simulink model "common_2"  (R2018b)
settings: Solver=ode4  StartTime=0.0  StopTime=tmax  FixedStep=0.005  RelTol=1e-3  EnableMultiTasking=on
values from neighbouring files (symbols this model uses):
  dq_init = [0.01 0.01]    [paraInit.m]
  g = 9.81    [paraInit.m]
  q_init = [0.01 0.01]    [paraInit.m]
undefined symbols (not defined in the file or in its folder): para
settings Model: Creator=Administrator  LastModifiedBy=q5461
settings DataIOCC: LimitDataPoints=on
settings OptimizationCC: LifeSpan=inf
settings DebuggingCC: AllowSymbolicDim=off  SFUnexpectedBacktrackingDiag=warning  SFNoUnconditionalDefaultTransitionDiag=warning  SFExecutionAtInitializationDiag=none
settings ModelReferenceCC: PropagateSignalLabelsOutOfModel=off
settings SFSimCC: SimUseLocalCustomCode=off
settings RTWCC: RTWUseLocalCustomCode=off
settings CodeAppCC: StateflowObjectComments=on
settings GRTTargetCC: TargetLangStandard=C89/C90 (ANSI)
settings ConfigComp: CovMetricSettings=dw  CovHtmlReporting=on  CovSaveCumulativeToWorkspaceVar=on  CovSaveSingleToWorkspaceVar=on  CovExternalEMLEnable=off

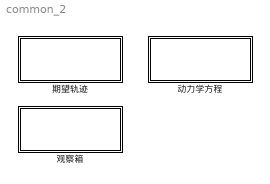
== system common_2 ==
  动力学方程 : Subsystem
  期望轨迹 : Subsystem
  观察箱 : Subsystem

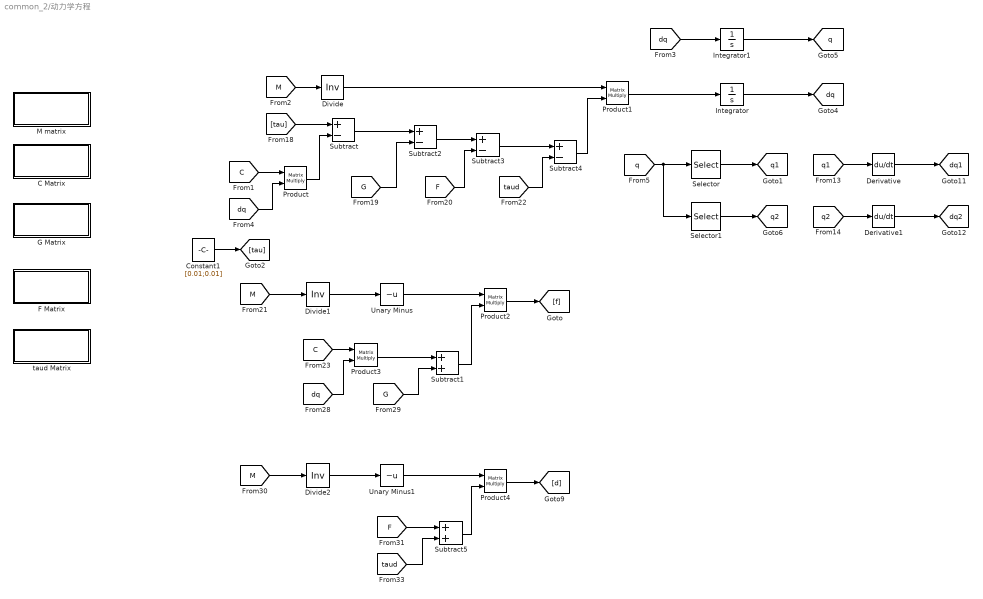
== system common_2/动力学方程 ==
  C Matrix : Subsystem
  Constant1 : Constant  Value=[0.01;0.01]
  Derivative : Derivative
  Derivative1 : Derivative
  Divide : Product  Inputs=/  Multiplication=Matrix(*)
  Divide1 : Product  Inputs=/  Multiplication=Matrix(*)
  Divide2 : Product  Inputs=/  Multiplication=Matrix(*)
  F Matrix : Subsystem
  G Matrix : Subsystem
  Integrator : Integrator  InitialCondition=dq_init
  Integrator1 : Integrator  InitialCondition=q_init
  M matrix : Subsystem
  Product{,1..4} (5 alike) : Product  Multiplication=Matrix(*)
  Selector : Selector  InputPortWidth=2  IndexOptions=Index vector (dialog)  Indices=[1]  OutputSizes=1
  Selector1 : Selector  InputPortWidth=2  IndexOptions=Index vector (dialog)  Indices=[2]  OutputSizes=1
  Subtract{,2..4} (4 alike) : Sum  Inputs=+-
  Subtract1 : Sum
  Subtract5 : Sum
  Unary Minus : UnaryMinus
  Unary Minus1 : UnaryMinus
  taud Matrix : Subsystem
  tag scope: dq1=global, dq2=global, dq=global, q1=global, q2=global, q=global
  wires:
  Integrator/1 -> [dq]
  [dq] -> Integrator1/1
  Integrator1/1 -> [q]
  Selector/1 -> [q1]
  Selector1/1 -> [q2]
  [q] -> Selector1/1, Selector/1
  [q1] -> Derivative/1
  Derivative/1 -> [dq1]
  [q2] -> Derivative1/1
  Derivative1/1 -> [dq2]
  [M] -> Divide/1
  Product1/1 -> Integrator/1
  Divide/1 -> Product1/1
  [tau] -> Subtract/1
  [C] -> Product/1
  [dq] -> Product/2
  Product/1 -> Subtract/2
  Subtract/1 -> Subtract2/1
  [G] -> Subtract2/2
  Subtract2/1 -> Subtract3/1
  [F] -> Subtract3/2
  Subtract3/1 -> Subtract4/1
  Subtract4/1 -> Product1/2
  [M] -> Divide1/1
  Divide1/1 -> Unary Minus/1
  Unary Minus/1 -> Product2/1
  [C] -> Product3/1
  [dq] -> Product3/2
  Product3/1 -> Subtract1/1
  [G] -> Subtract1/2
  Subtract1/1 -> Product2/2
  Product2/1 -> [f]
  [M] -> Divide2/1
  Divide2/1 -> Unary Minus1/1
  Unary Minus1/1 -> Product4/1
  [F] -> Subtract5/1
  [taud] -> Subtract5/2
  Subtract5/1 -> Product4/2
  Product4/1 -> [d]
  Constant1/1 -> [tau]
  [taud] -> Subtract4/2

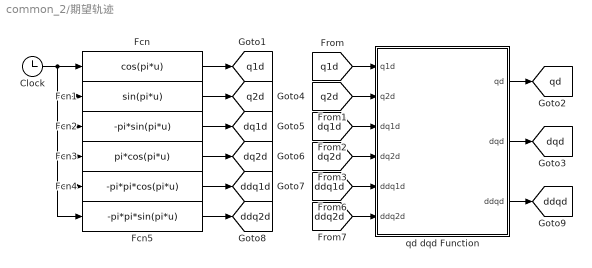
== system common_2/期望轨迹 ==
  Clock : Clock
  Fcn : Fcn  Expr=cos(pi*u)
  Fcn1 : Fcn  Expr=sin(pi*u)
  Fcn2 : Fcn  Expr=-pi*sin(pi*u)
  Fcn3 : Fcn  Expr=pi*cos(pi*u)
  Fcn4 : Fcn  Expr=-pi*pi*cos(pi*u)
  Fcn5 : Fcn  Expr=-pi*pi*sin(pi*u)
  qd dqd Function : MATLAB Function  TreatAsAtomicUnit=on
  tag scope: ddq1d=global, ddq2d=global, ddqd=global, dq1d=global, dq2d=global, dqd=global, q1d=global, q2d=global, qd=global
  wires:
  qd dqd Function/2(dqd) -> [dqd]
  qd dqd Function/1(qd) -> [qd]
  Clock/1 -> Fcn5/1, Fcn4/1, Fcn3/1, Fcn2/1, Fcn1/1, Fcn/1
  Fcn/1 -> [q1d]
  Fcn1/1 -> [q2d]
  Fcn2/1 -> [dq1d]
  Fcn3/1 -> [dq2d]
  [q1d] -> qd dqd Function/1(q1d)
  [q2d] -> qd dqd Function/2(q2d)
  [dq1d] -> qd dqd Function/3(dq1d)
  [dq2d] -> qd dqd Function/4(dq2d)
  Fcn4/1 -> [ddq1d]
  [ddq1d] -> qd dqd Function/5(ddq1d)
  [ddq2d] -> qd dqd Function/6(ddq2d)
  qd dqd Function/3(ddqd) -> [ddqd]
  Fcn5/1 -> [ddq2d]

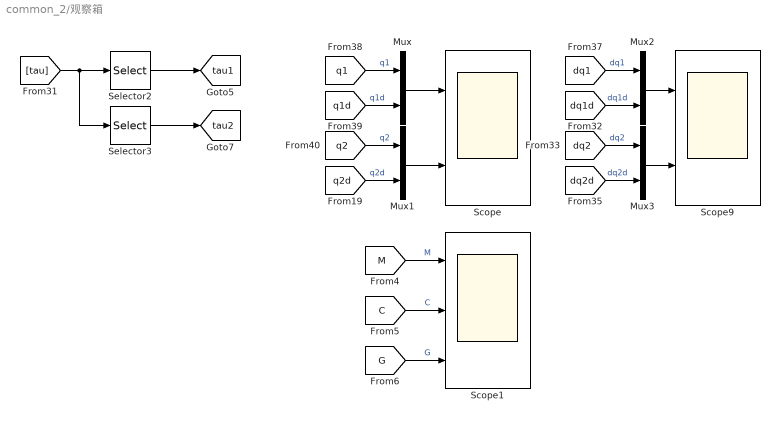
== system common_2/观察箱 ==
  Mux{,1..3} (4 alike) : Mux  Inputs=2
  Scope : Scope  NumInputPorts=2
  Scope1 : Scope  NumInputPorts=3
  Scope9 : Scope  NumInputPorts=2
  Selector2 : Selector  InputPortWidth=2  IndexOptions=Index vector (dialog)  Indices=[1]  OutputSizes=1
  Selector3 : Selector  InputPortWidth=2  IndexOptions=Index vector (dialog)  Indices=[2]  OutputSizes=1
  tag scope: tau1=global, tau2=global
  wires:
  [q1] -> Mux/1  "q1"
  [q1d] -> Mux/2  "q1d"
  Mux/1 -> Scope/1
  [q2] -> Mux1/1  "q2"
  [q2d] -> Mux1/2  "q2d"
  Mux1/1 -> Scope/2
  [dq1] -> Mux2/1  "dq1"
  [dq1d] -> Mux2/2  "dq1d"
  Mux2/1 -> Scope9/1
  [dq2] -> Mux3/1  "dq2"
  [dq2d] -> Mux3/2  "dq2d"
  Mux3/1 -> Scope9/2
  Selector2/1 -> [tau1]
  Selector3/1 -> [tau2]
  [tau] -> Selector3/1, Selector2/1
  [M] -> Scope1/1  "M"
  [C] -> Scope1/2  "C"
  [G] -> Scope1/3  "G"

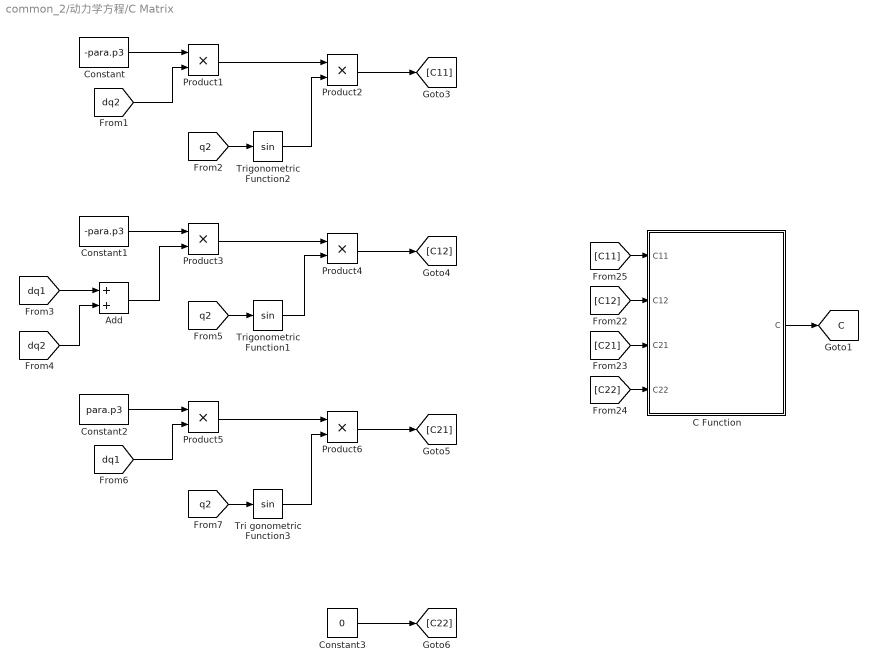
== system common_2/动力学方程/C Matrix ==
  Add : Sum
  C Function : MATLAB Function  TreatAsAtomicUnit=on
  Constant : Constant  Value=-para.p3
  Constant1 : Constant  Value=-para.p3
  Constant2 : Constant  Value=para.p3
  Constant3 : Constant  Value=0
  Product{1..6} (6 alike) : Product
  Tri gonometric Function3 : Trigonometry
  Trigonometric Function1 : Trigonometry
  Trigonometric Function2 : Trigonometry
  tag scope: C=global
  wires:
  [dq2] -> Product1/2
  Constant3/1 -> [C22]
  [q2] -> Tri gonometric Function3/1
  [q2] -> Trigonometric Function1/1
  Product6/1 -> [C21]
  Product3/1 -> Product4/1
  [C12] -> C Function/2(C12)
  Tri gonometric Function3/1 -> Product6/2
  Trigonometric Function1/1 -> Product4/2
  [dq2] -> Add/2
  Constant2/1 -> Product5/1
  Product5/1 -> Product6/1
  [C11] -> C Function/1(C11)
  C Function/1(C) -> [C]
  [q2] -> Trigonometric Function2/1
  Constant/1 -> Product1/1
  Product1/1 -> Product2/1
  [C22] -> C Function/4(C22)
  Product4/1 -> [C12]
  Product2/1 -> [C11]
  Trigonometric Function2/1 -> Product2/2
  [C21] -> C Function/3(C21)
  [dq1] -> Product5/2
  Constant1/1 -> Product3/1
  Add/1 -> Product3/2
  [dq1] -> Add/1

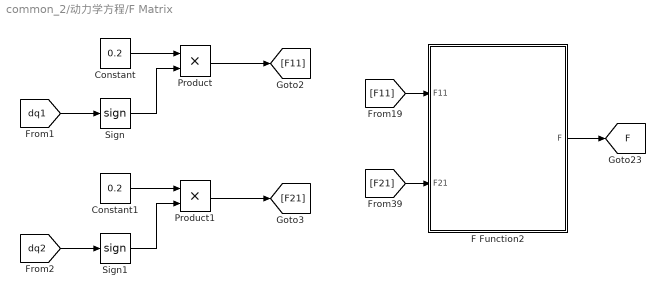
== system common_2/动力学方程/F Matrix ==
  Constant : Constant  Value=0.2
  Constant1 : Constant  Value=0.2
  F Function2 : MATLAB Function  TreatAsAtomicUnit=on
  Product : Product
  Product1 : Product
  Sign : Signum
  Sign1 : Signum
  tag scope: F=global
  wires:
  Sign1/1 -> Product1/2
  Product1/1 -> [F21]
  [dq2] -> Sign1/1
  Constant1/1 -> Product1/1
  [dq1] -> Sign/1
  Product/1 -> [F11]
  Sign/1 -> Product/2
  F Function2/1(F) -> [F]
  Constant/1 -> Product/1
  [F21] -> F Function2/2(F21)
  [F11] -> F Function2/1(F11)

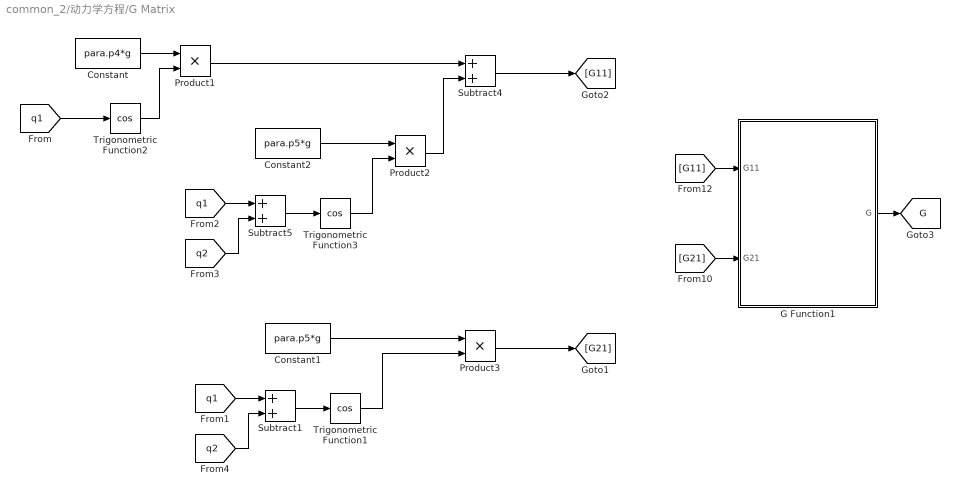
== system common_2/动力学方程/G Matrix ==
  Constant : Constant  Value=para.p4*g
  Constant1 : Constant  Value=para.p5*g
  Constant2 : Constant  Value=para.p5*g
  G Function1 : MATLAB Function  TreatAsAtomicUnit=on
  Product1 : Product
  Product2 : Product
  Product3 : Product
  Subtract1 : Sum
  Subtract4 : Sum
  Subtract5 : Sum
  Trigonometric Function1 : Trigonometry  Operator=cos
  Trigonometric Function2 : Trigonometry  Operator=cos
  Trigonometric Function3 : Trigonometry  Operator=cos
  tag scope: G=global
  wires:
  Product2/1 -> Subtract4/2
  [q1] -> Subtract1/1
  Subtract4/1 -> [G11]
  Subtract1/1 -> Trigonometric Function1/1
  Trigonometric Function2/1 -> Product1/2
  [q1] -> Subtract5/1
  Constant1/1 -> Product3/1
  [q2] -> Subtract5/2
  Trigonometric Function1/1 -> Product3/2
  [q2] -> Subtract1/2
  Trigonometric Function3/1 -> Product2/2
  Constant/1 -> Product1/1
  Constant2/1 -> Product2/1
  G Function1/1(G) -> [G]
  Product1/1 -> Subtract4/1
  Product3/1 -> [G21]
  Subtract5/1 -> Trigonometric Function3/1
  [G11] -> G Function1/1(G11)
  [q1] -> Trigonometric Function2/1
  [G21] -> G Function1/2(G21)

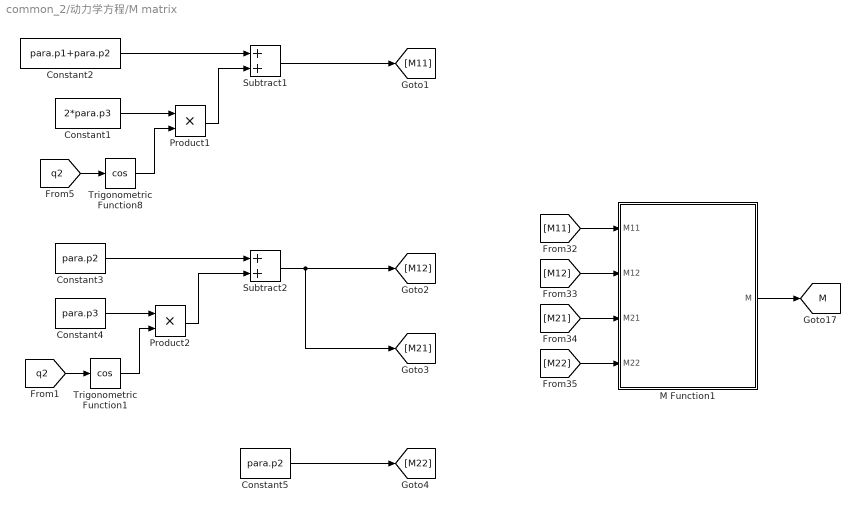
== system common_2/动力学方程/M matrix ==
  Constant1 : Constant  Value=2*para.p3
  Constant2 : Constant  Value=para.p1+para.p2
  Constant3 : Constant  Value=para.p2
  Constant4 : Constant  Value=para.p3
  Constant5 : Constant  Value=para.p2
  M Function1 : MATLAB Function  TreatAsAtomicUnit=on
  Product1 : Product
  Product2 : Product
  Subtract1 : Sum
  Subtract2 : Sum
  Trigonometric Function1 : Trigonometry  Operator=cos
  Trigonometric Function8 : Trigonometry  Operator=cos
  tag scope: M=global
  wires:
  Trigonometric Function1/1 -> Product2/2
  Subtract1/1 -> [M11]
  [q2] -> Trigonometric Function1/1
  [M22] -> M Function1/4(M22)
  Constant5/1 -> [M22]
  Constant4/1 -> Product2/1
  Constant1/1 -> Product1/1
  [M21] -> M Function1/3(M21)
  Subtract2/1 -> [M21], [M12]
  Trigonometric Function8/1 -> Product1/2
  M Function1/1(M) -> [M]
  [M11] -> M Function1/1(M11)
  Constant3/1 -> Subtract2/1
  [M12] -> M Function1/2(M12)
  Product1/1 -> Subtract1/2
  Constant2/1 -> Subtract1/1
  [q2] -> Trigonometric Function8/1
  Product2/1 -> Subtract2/2

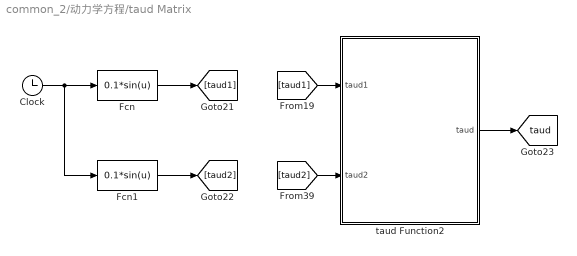
== system common_2/动力学方程/taud Matrix ==
  Clock : Clock
  Fcn : Fcn  Expr=0.1*sin(u)
  Fcn1 : Fcn  Expr=0.1*sin(u)
  taud Function2 : MATLAB Function  TreatAsAtomicUnit=on
  tag scope: taud=global
  wires:
  [taud1] -> taud Function2/1(taud1)
  Fcn/1 -> [taud1]
  Fcn1/1 -> [taud2]
  taud Function2/1(taud) -> [taud]
  Clock/1 -> Fcn1/1, Fcn/1
  [taud2] -> taud Function2/2(taud2)

== matlab function common_2/期望轨迹/qd dqd Function ==
  data: q1d input; qd output; q2d input; dq1d input; dq2d input; dqd output; ddq1d input; ddq2d input; ddqd output
function [qd,dqd,ddqd]= fcn(q1d,q2d,dq1d,dq2d,ddq1d,ddq2d)
%#codegen

qd   = [q1d;q2d];
dqd  = [dq1d;dq2d];
ddqd = [ddq1d;ddq2d];

== matlab function common_2/动力学方程/G Matrix/G Function1 ==
  data: G11 input; G output; G21 input
function G = fcn(G11,G21)
%#codegen

G = [G11;G21];

== matlab function common_2/动力学方程/C Matrix/C Function ==
  data: C11 input; C output; C12 input; C21 input; C22 input
function C = fcn(C11,C12,C21,C22)
%#codegen

C = [C11 C12;C21 C22];

== matlab function common_2/动力学方程/M matrix/M Function1 ==
  data: M11 input; M output; M12 input; M21 input; M22 input
function M = fcn(M11,M12,M21,M22)
%#codegen

M = [M11 M12;M21 M22];

== matlab function common_2/动力学方程/F Matrix/F Function2 ==
  data: F11 input; F output; F21 input
function F = fcn(F11,F21)
%#codegen

F = [F11;F21];

== matlab function common_2/动力学方程/taud Matrix/taud Function2 ==
  data: taud1 input; taud output; taud2 input
function taud = fcn(taud1,taud2)
%#codegen

taud = [taud1;taud2];
